simulink model "InvPendCont"  (Simulink 7.7)
settings: Solver=ode45  StartTime=0.0  StopTime=2  FixedStep=0.001  RelTol=1e-3
values from neighbouring files (symbols this model uses):
  A = [0 1;g/L 0]    [setupInvPend.m]
  amp = pi/6    (= 0.523598775598)    [setupInvPend.m]
  b = [0;1/J]    [setupInvPend.m]
  c = [1 0]    [setupInvPend.m]
  K1 = 5*J+g*J/L    (= 74.4)    [setupInvPend.m]
  K2 = 4*J    (= 36)    [setupInvPend.m]
  Kd = 1749    [setupInvPend.m]    (also in setupPID.m = 2.56637061436)
  Ki = 0    [setupInvPend.m]    (also in setupPID.m = 4961.00426885)
  Kp = 85000    [setupInvPend.m]    (also in setupPID.m = 394.784176044)
  omega = 10    [setupInvPend.m]    (also in setupPID.m = 62.8318530718)
  phi = pi/8    (= 0.392699081699)    [setupInvPend.m]
libraries: simulink x1
settings Model: Creator=Rob  LastModifiedBy=rjwood
settings OptimizationCC: InitFltsAndDblsToZero=on
settings DebuggingCC: SaveWithParameterizedLinksMsg=none  SignalResolutionControl=TryResolveAllWithWarning  StrictBusMsg=Warning
settings GRTTargetCC: TargetFcnLib=ansi_tfl_tmw.mat

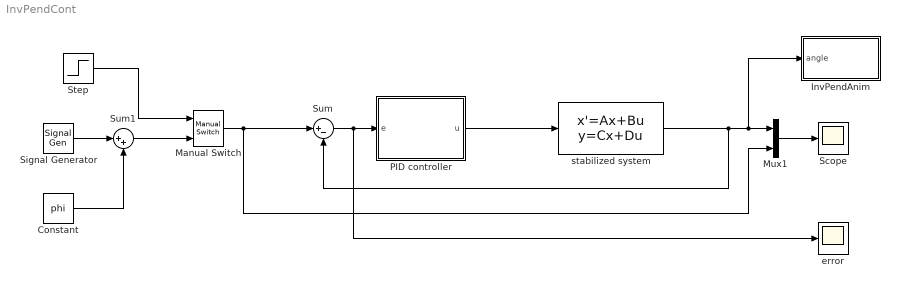
== system InvPendCont ==
  Constant : Constant  Value=phi
  InvPendAnim : Subsystem
  Manual Switch : simulink/Signal Routing/Manual Switch  SystemSampleTime=-1  sw=1  action=0  varsize=off
  Mux1 : Mux  Inputs=2
  PID controller : Subsystem
  Scope : Scope
      settings: YMin=0.1  YMax=1.05
  Signal Generator : SignalGenerator  WaveForm=square  Amplitude=amp  Frequency=omega  Units=rad/sec
  Step : Step  Time=0  SampleTime=0
  Sum : Sum  Inputs=|+-
  Sum1 : Sum  Inputs=|++
  error : Scope
      settings: YMin=-0.009  YMax=0.009
  stabilized system : StateSpace  A=A-b*[K1 K2]  B=b  C=c  D=0
  wires:
  Mux1/1 -> Scope/1
  stabilized system/1 -> Sum/2, Mux1/1, InvPendAnim/1(angle)
  Manual Switch/1 -> Mux1/2, Sum/1
  Sum1/1 -> Manual Switch/2
  Step/1 -> Manual Switch/1
  Sum/1 -> PID controller/1(e), error/1
  PID controller/1(u) -> stabilized system/1
  Signal Generator/1 -> Sum1/1
  Constant/1 -> Sum1/2

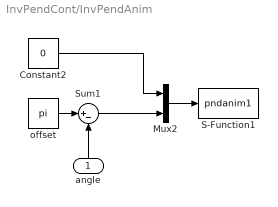
== system InvPendCont/InvPendAnim ==
  angle : Inport
  Constant2 : Constant  Value=0
  Mux2 : Mux  Inputs=2
  S-Function1 : S-Function  FunctionName=pndanim1  Parameters=0.001  EnableBusSupport=off
  Sum1 : Sum  Inputs=|+-
  offset : Constant  Value=pi
  wires:
  Mux2/1 -> S-Function1/1
  Constant2/1 -> Mux2/1
  offset/1 -> Sum1/1
  Sum1/1 -> Mux2/2
  angle/1 -> Sum1/2

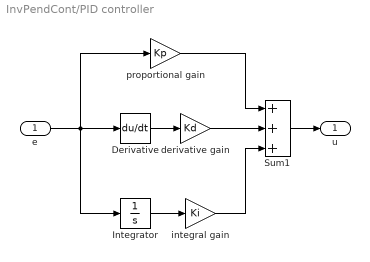
== system InvPendCont/PID controller ==
  e : Inport
  Derivative : Derivative
  Integrator : Integrator
  Sum1 : Sum  Inputs=+++
  derivative gain : Gain  Gain=Kd
  integral gain : Gain  Gain=Ki
  proportional gain : Gain  Gain=Kp
  u : Outport
  wires:
  integral gain/1 -> Sum1/3
  Integrator/1 -> integral gain/1
  Sum1/1 -> u/1
  derivative gain/1 -> Sum1/2
  proportional gain/1 -> Sum1/1
  Derivative/1 -> derivative gain/1
  e/1 -> Integrator/1, Derivative/1, proportional gain/1
